simulink model "WindTurbine_FullPlant"  (R2025a)
settings: Solver=VariableStepAuto  StartTime=0.0  StopTime=20  RelTol=1e-3
settings Model: Creator=hero  LastModifiedBy=hero

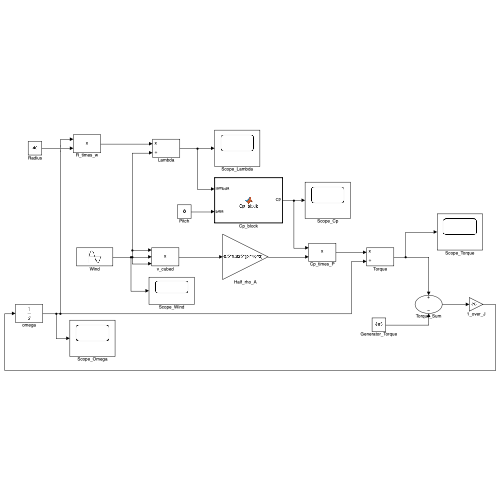
[thumbnail: Simulink's stored preview of the top-level diagram]
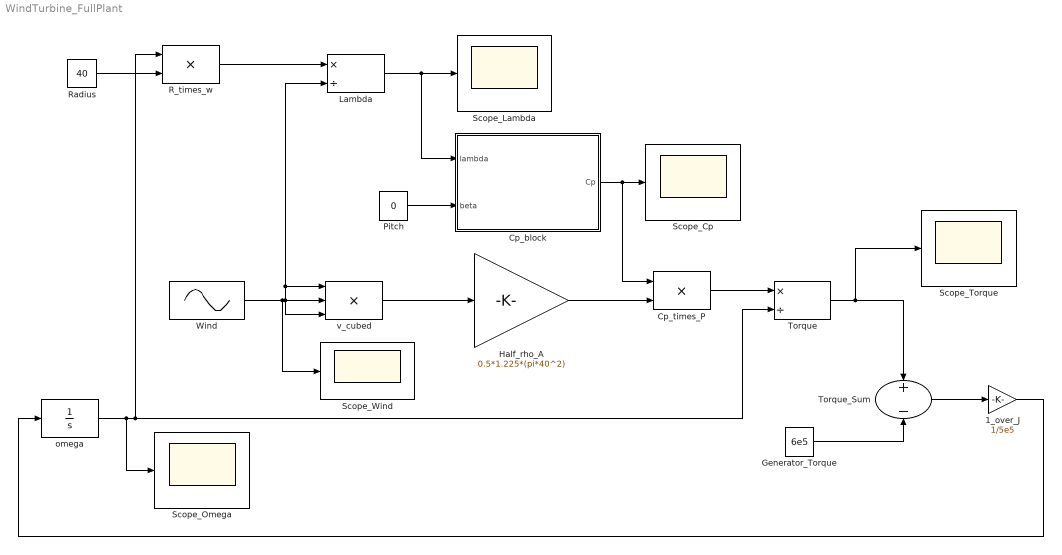
== system WindTurbine_FullPlant ==
  1_over_J : Gain  Gain=1/5e5
  Cp_block : MATLAB Function  TreatAsAtomicUnit=on
  Cp_times_P : Product
  Generator_Torque : Constant  Value=6e5
  Half_rho_A : Gain  Gain=0.5*1.225*(pi*40^2)
  Lambda : Product  Inputs=*/
  Pitch : Constant  Value=0
  R_times_w : Product
  Radius : Constant  Value=40
  Scope_Cp : Scope
  Scope_Lambda : Scope
  Scope_Omega : Scope
  Scope_Torque : Scope
  Scope_Wind : Scope
  Torque : Product  Inputs=*/
  Torque_Sum : Sum  Inputs=+-
  Wind : Sin  Amplitude=2  Bias=10  Frequency=0.3  SampleTime=0
  omega : Integrator  InitialCondition=1
  v_cubed : Product  Inputs=3
  wires:
  1_over_J/1 -> omega/1
  Torque_Sum/1 -> 1_over_J/1
  Half_rho_A/1 -> Cp_times_P/2
  Lambda/1 -> Cp_block/1(lambda), Scope_Lambda/1
  Torque/1 -> Scope_Torque/1, Torque_Sum/1
  Wind/1 -> v_cubed/1, Lambda/2, v_cubed/3, v_cubed/2, Scope_Wind/1
  Cp_block/1(Cp) -> Cp_times_P/1, Scope_Cp/1
  R_times_w/1 -> Lambda/1
  Generator_Torque/1 -> Torque_Sum/2
  v_cubed/1 -> Half_rho_A/1
  Cp_times_P/1 -> Torque/1
  Pitch/1 -> Cp_block/2(beta)
  omega/1 -> R_times_w/1, Torque/2, Scope_Omega/1
  Radius/1 -> R_times_w/2

== matlab function WindTurbine_FullPlant/Cp_block ==
  data: lambda input; Cp output; beta input
function Cp = Cp_block(lambda,beta)
lambda_i = 1/((1/(lambda+0.08*beta))-(0.035/(beta^3+1)));
Cp = 0.22*((116/lambda_i)-0.4*beta-5)*exp(-12.5/lambda_i);
end
